simulink model "prop1"  (R2015a)
settings: Solver=ode45  StartTime=0.0  StopTime=10.0  RelTol=1e-3
libraries: simulink x5
settings Model: Creator=teme  LastModifiedBy=teme

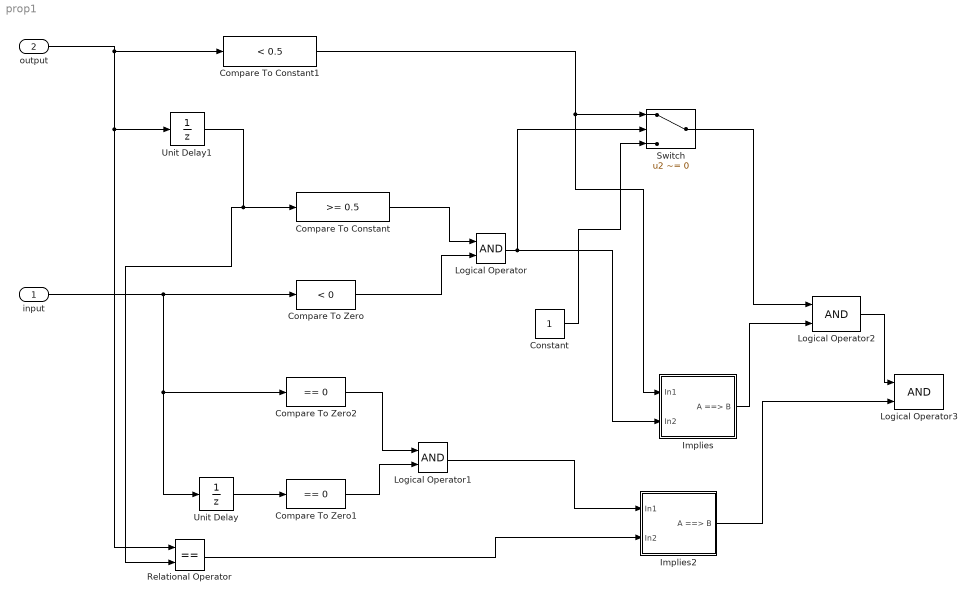
== system prop1 ==
  input : Inport
  output : Inport  Port=2
  Compare To Constant : simulink/Logic and Bit Operations/Compare To Constant  relop=>=  const=0.5  OutDataTypeStr=boolean
  Compare To Constant1 : simulink/Logic and Bit Operations/Compare To Constant  relop=<  const=0.5  OutDataTypeStr=boolean
  Compare To Zero : simulink/Logic and Bit Operations/Compare To Zero  relop=<  OutDataTypeStr=boolean
  Compare To Zero1 : simulink/Logic and Bit Operations/Compare To Zero  relop===  OutDataTypeStr=boolean
  Compare To Zero2 : simulink/Logic and Bit Operations/Compare To Zero  relop===  OutDataTypeStr=boolean
  Constant : Constant
  Implies : Subsystem  TreatAsAtomicUnit=on  mask(Implies){}
  Implies2 : Subsystem  TreatAsAtomicUnit=on
  Logical Operator{,1..3} (4 alike) : Logic  AllPortsSameDT=off  OutDataTypeStr=boolean
  Relational Operator : RelationalOperator  Operator===  OutDataTypeStr=boolean
  Switch : Switch  Criteria=u2 ~= 0
  Unit Delay : UnitDelay  SampleTime=-1
  Unit Delay1 : UnitDelay  SampleTime=-1
  wires:
  input/1 -> Unit Delay/1, Compare To Zero2/1, Compare To Zero/1
  Compare To Constant/1 -> Logical Operator/1
  Compare To Zero/1 -> Logical Operator/2
  Logical Operator/1 -> Implies/2(In2), Switch/2
  Constant/1 -> Switch/3
  output/1 -> Compare To Constant1/1, Relational Operator/1, Unit Delay1/1
  Compare To Constant1/1 -> Implies/1(In1), Switch/1
  Unit Delay/1 -> Compare To Zero1/1
  Compare To Zero2/1 -> Logical Operator1/1
  Compare To Zero1/1 -> Logical Operator1/2
  Logical Operator1/1 -> Implies2/1(In1)
  Unit Delay1/1 -> Relational Operator/2, Compare To Constant/1
  Relational Operator/1 -> Implies2/2(In2)
  Implies2/1(A ==> B) -> Logical Operator3/2
  Switch/1 -> Logical Operator2/1
  Logical Operator2/1 -> Logical Operator3/1
  Implies/1(A ==> B) -> Logical Operator2/2

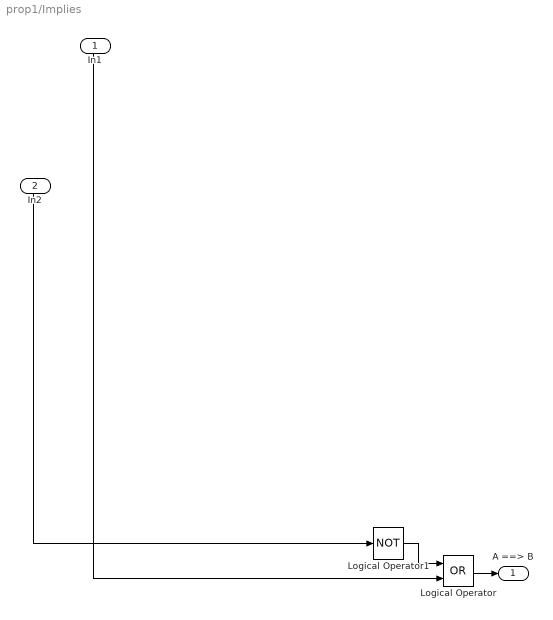
== system prop1/Implies ==
  In1 : Inport
  In2 : Inport  Port=2
  Logical Operator : Logic  Operator=OR  AllPortsSameDT=off  OutDataTypeStr=boolean
  Logical Operator1 : Logic  Operator=NOT  AllPortsSameDT=off  OutDataTypeStr=boolean
  A ==> B : Outport
  wires:
  Logical Operator1/1 -> Logical Operator/1
  In2/1 -> Logical Operator1/1
  In1/1 -> Logical Operator/2
  Logical Operator/1 -> A ==> B/1

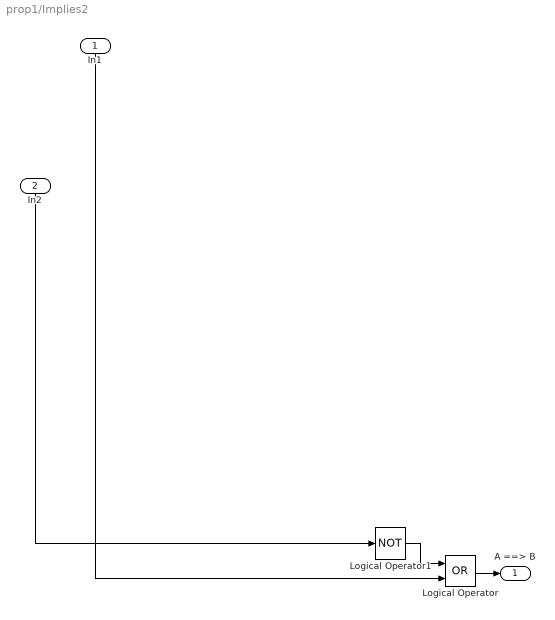
== system prop1/Implies2 ==
  In1 : Inport
  In2 : Inport  Port=2
  Logical Operator : Logic  Operator=OR  AllPortsSameDT=off  OutDataTypeStr=boolean
  Logical Operator1 : Logic  Operator=NOT  AllPortsSameDT=off  OutDataTypeStr=boolean
  A ==> B : Outport
  wires:
  Logical Operator1/1 -> Logical Operator/1
  In2/1 -> Logical Operator1/1
  In1/1 -> Logical Operator/2
  Logical Operator/1 -> A ==> B/1
